simulink model "a2e2"  (R2020a)
settings: Solver=FixedStepAuto  StartTime=0.0  StopTime=400000  FixedStep=0.01  RelTol=1e-3
settings Model: EnablePacing=on  PacingRate=6  Creator=mumun  LastModifiedBy=mumun

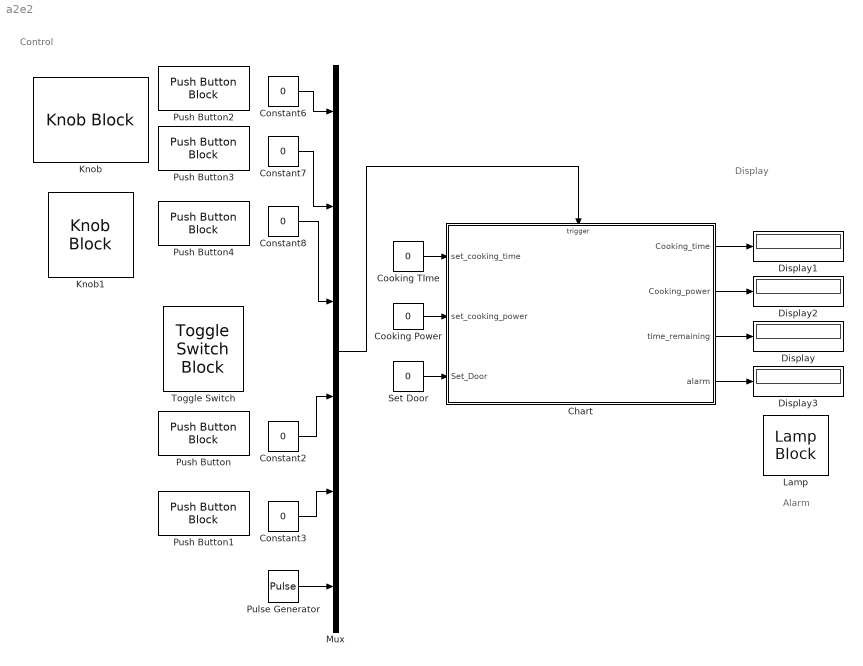
== system a2e2 ==
  note: Display
  note: Control
  note: Alarm
  Chart : Stateflow chart  TreatAsAtomicUnit=on
  Constant{2..3,6..8} (5 alike) : Constant  Value=0
  Cooking Power : Constant  Value=0  OutDataTypeStr=int64
  Cooking TIme : Constant  Value=0  OutMin=[0]  OutMax=[1000]  OutDataTypeStr=int64
  Display{,1..3} (4 alike) : Display
  Knob : KnobBlock  ScaleMax=1000
  Knob1 : KnobBlock  ScaleMax=800
  Lamp : LampBlock  LabelPosition=Hide
  Mux : Mux  Inputs=6
  Pulse Generator : DiscretePulseGenerator  PulseType=Time based  Period=1  PulseWidth=90
  Push Button : PushButtonBlock  ButtonText=Start_cooking
  Push Button1 : PushButtonBlock  ButtonText=Stop
  Push Button2 : PushButtonBlock  ButtonText=Turn_on
  Push Button3 : PushButtonBlock  ButtonText=set_time
  Push Button4 : PushButtonBlock  ButtonText=set_power
  Set Door : Constant  Value=0
  Toggle Switch : ToggleSwitchBlock
      settings: Values={{'open', 'Close'}, [0 1]}
  wires:
  Mux/1 -> Chart/Trigger
  Constant2/1 -> Mux/4
  Constant3/1 -> Mux/5
  Pulse Generator/1 -> Mux/6
  Constant6/1 -> Mux/1
  Cooking TIme/1 -> Chart/1(set_cooking_time)
  Cooking Power/1 -> Chart/2(set_cooking_power)
  Constant8/1 -> Mux/3
  Constant7/1 -> Mux/2
  Chart/3(time_remaining) -> Display/1
  Chart/1(Cooking_time) -> Display1/1
  Chart/2(Cooking_power) -> Display2/1
  Set Door/1 -> Chart/3(Set_Door)
  Chart/4(alarm) -> Display3/1

== stateflow chart a2e2/Chart ==
  settings: executeAtInitialization=1
  state Timer
    en:Idle_time=0;
    on pulse: time_counter();
    state Idle
      en:Cooking_time=0;Cooking_power=0;
      en: time_count=0;time_remaining=0;
      en: alarm=0;
    state cooking_time_power
      en:Idle_time=0;
      on set_time:Cooking_time= set_cooking_time;
      on set_power:Cooking_power= set_cooking_power
    state door_close
      en:Idle_time=0;
    state start_cooking
      en: time_remaining = 1;
      on pulse: increase_time();
      du:  time_remaining=  Cooking_time - time_count;
      on set_time:Cooking_time= set_cooking_time;
      on set_power:Cooking_power= set_cooking_power
    state Cooking_finish
      en:Cooking_time=0;Cooking_power=0;
      en: time_count=0;time_remaining=0;
      en: alarm=1;
    state suspend_cooking
    cooking_time_power -> Idle [order 3] : [Idle_time>300]
    cooking_time_power -> door_close [order 1] : [Set_Door==1]
    (default) -> Idle
    door_close -> cooking_time_power [order 2] : [Set_Door==0]
    Idle -> cooking_time_power : Turn_on
    suspend_cooking -> door_close [order 1] : [Set_Door==1]
    cooking_time_power -> Idle [order 2] : Stop
    Cooking_finish -> Idle : Stop
    door_close -> Idle [order 3] : Stop
    suspend_cooking -> Idle [order 2] : Stop
    door_close -> Idle [order 4] : [Idle_time>300]
    door_close -> start_cooking [order 1] : Start_cooking
    start_cooking -> Cooking_finish [order 4] : [set_cooking_time==0||set_cooking_power==0]
    start_cooking -> Cooking_finish [order 3] : [time_remaining<1]
    start_cooking -> suspend_cooking [order 2] : [Set_Door==0]
    start_cooking -> suspend_cooking [order 1] : Stop
  (default) -> Timer
  data: Cooking_time output int64; set_cooking_time input; set_cooking_power input; Cooking_power output int64; time_remaining output int64; time_count local int64; Set_Door input; Idle_time local; alarm output
  events: Turn_on input RISING_EDGE_EVENT; set_time input RISING_EDGE_EVENT; set_power input RISING_EDGE_EVENT; Start_cooking input RISING_EDGE_EVENT; Stop input RISING_EDGE_EVENT; pulse input RISING_EDGE_EVENT
  function time_counter:
    | function time_counter
    | Idle_time =(Idle_time+1);
    | 
    | end
  function increase_time:
    | function increase_time
    | time_count =(time_count+1);
    | 
    | end
